simulink library "powerlib_models"  (Simulink 6.0)
settings: Solver=ode45  SolverMode=SingleTasking  StartTime=0.0  StopTime=10.0  RelTol=1e-3
values from neighbouring files (symbols this model uses):
  Ts = get(handles.edit1,'string')    [powergui.m]
undefined symbols (not defined in the file or in its folder): A, a0, a1, a2, a3, a4, a5, Ac, Amplitude, Amplitudes, B, BaseCurrent, BaseFlux, Bc, C, Capacitance, Cc, Columns, ConnectionType, Cs, ctrl, current, Current, damp, Dc, Dd, DiscIntNeverNeededParam, dref, dwo, exc, excAxis, F, Flux, fnom, Frequency, FreqVps, Gain1, gate, GH, GHd, GI, GId, GL, GLd, H, HarmonicGeneration, HT, hyd, I1_init, ib, ib2, Id1o, Inductance, InitialFlux, InitialSlope, io, Iq1o, isfinite, j, J ... (+138)
libraries: powerlib_models x32, powerlib_extras x4
(part 8 of 11)

== system powerlib_models/Discrete/asynchronous_machine/Rotor ==
  vqr,vdr : Inport  Port=1  LatchInput=off
  w-wr : Inport  Port=2  LatchInput=off
  phimq,phimd : Inport  Port=3  LatchInput=off
  1\Llr : Gain  Gain=1/Llr  SaturateOnIntegerOverflow=on
  1\Llr1 : Gain  Gain=Rr  SaturateOnIntegerOverflow=on
  1\Llr2 : Gain  Gain=1/Llr  SaturateOnIntegerOverflow=on
  1\Llr3 : Gain  Gain=Rr  SaturateOnIntegerOverflow=on
  Demux : Demux  Outputs=2
  Demux1 : Demux  Outputs=2
  Discrete-Time Integrator : DiscreteIntegrator  InitialCondition=phirqo  SampleTime=Ts  ICPrevOutput=DiscIntNeverNeededParam  ICPrevScaledInput=DiscIntNeverNeededParam
  Discrete-Time Integrator1 : DiscreteIntegrator  InitialCondition=phirdo  SampleTime=Ts  ICPrevOutput=DiscIntNeverNeededParam  ICPrevScaledInput=DiscIntNeverNeededParam
  Mux2 : Mux  Inputs=2
  Mux3 : Mux  Inputs=2
  Product : Product  SaturateOnIntegerOverflow=on  InputSameDT=on
  Product1 : Product  Orientation=left  SaturateOnIntegerOverflow=on  InputSameDT=on
  Sum1 : Sum  Inputs=++-||  SaturateOnIntegerOverflow=on  InputSameDT=on
  Sum2 : Sum  Inputs=+--  SaturateOnIntegerOverflow=on  InputSameDT=on
  Sum3 : Sum  Inputs=+-|  SaturateOnIntegerOverflow=on  InputSameDT=on
  Sum4 : Sum  Inputs=-+|  SaturateOnIntegerOverflow=on  InputSameDT=on
  web1 : Gain  Gain=web_psb  SaturateOnIntegerOverflow=on
  web_psb : Gain  Gain=web_psb  SaturateOnIntegerOverflow=on
  iqr,idr : Outport
  phiqr,phidr : Outport  Port=2
  wires:
  Mux3/1 -> phiqr,phidr/1
  Discrete-Time Integrator/1 -> Mux3/1, Product1/2, Sum3/1  "phiqr"
  web1/1 -> Discrete-Time Integrator1/1
  Sum1/1 -> web1/1
  w-wr/1 -> Product/2, Product1/1
  Product/1 -> Sum2/2
  web_psb/1 -> Discrete-Time Integrator/1
  Sum2/1 -> web_psb/1
  Discrete-Time Integrator1/1 -> Sum4/2, Product/1, Mux3/2
  vqr,vdr/1 -> Demux/1
  Product1/1 -> Sum1/1
  Demux/2 -> Sum1/2
  1\Llr3/1 -> Sum1/3
  1\Llr2/1 -> 1\Llr3/1, Mux2/2  "idr"
  Sum4/1 -> 1\Llr2/1
  Demux1/2 -> Sum4/1
  Mux2/1 -> iqr,idr/1
  1\Llr/1 -> Mux2/1, 1\Llr1/1  "iqr"
  1\Llr1/1 -> Sum2/3
  Sum3/1 -> 1\Llr/1
  Demux/1 -> Sum2/1
  Demux1/1 -> Sum3/2
  phimq,phimd/1 -> Demux1/1

== system powerlib_models/Discrete/asynchronous_machine/Stator ==
  phimq,phimd : Inport  Port=1  LatchInput=off
  vqs,vds : Inport  Port=2  LatchInput=off
  w : Inport  Port=3  LatchInput=off
  1\Llr : Gain  Gain=1/Lls  SaturateOnIntegerOverflow=on
  1\Llr1 : Gain  Gain=Rs  SaturateOnIntegerOverflow=on
  1\Llr2 : Gain  Gain=1/Lls  SaturateOnIntegerOverflow=on
  1\Llr3 : Gain  Gain=Rs  SaturateOnIntegerOverflow=on
  Demux : Demux  Outputs=2
  Demux1 : Demux  Outputs=2
  Discrete-Time Integrator : DiscreteIntegrator  InitialCondition=phisqo  SampleTime=Ts  ICPrevOutput=DiscIntNeverNeededParam  ICPrevScaledInput=DiscIntNeverNeededParam
  Discrete-Time Integrator1 : DiscreteIntegrator  InitialCondition=phisdo  SampleTime=Ts  ICPrevOutput=DiscIntNeverNeededParam  ICPrevScaledInput=DiscIntNeverNeededParam
  Mux2 : Mux  Inputs=2
  Mux3 : Mux  Inputs=2
  Mux4 : Mux  Inputs=2
  Product : Product  SaturateOnIntegerOverflow=on  InputSameDT=on
  Product1 : Product  SaturateOnIntegerOverflow=on  InputSameDT=on
  Sum1 : Sum  Inputs=++-||  SaturateOnIntegerOverflow=on  InputSameDT=on
  Sum2 : Sum  Inputs=--+  SaturateOnIntegerOverflow=on  InputSameDT=on
  Sum3 : Sum  Inputs=-+  SaturateOnIntegerOverflow=on  InputSameDT=on
  Sum4 : Sum  Inputs=+-|  SaturateOnIntegerOverflow=on  InputSameDT=on
  web1 : Gain  Gain=web_psb  SaturateOnIntegerOverflow=on
  web_psb : Gain  Gain=web_psb  SaturateOnIntegerOverflow=on
  phiqs,phids : Outport
  iqs,ids : Outport  Port=2
  phis,is : Outport  Port=3
  wires:
  phimq,phimd/1 -> Demux1/1
  Demux1/1 -> Sum4/2
  Sum4/1 -> 1\Llr/1
  1\Llr/1 -> Mux2/1, 1\Llr1/1  "iqs"
  1\Llr1/1 -> Sum2/1
  vqs,vds/1 -> Demux/1
  Sum2/1 -> web_psb/1
  Demux/1 -> Sum2/3
  Product/1 -> Sum2/2
  web_psb/1 -> Discrete-Time Integrator/1
  Discrete-Time Integrator/1 -> Mux3/1, Product1/2, Sum4/1
  Mux2/1 -> iqs,ids/1, Mux4/2
  w/1 -> Product/1, Product1/1
  Demux1/2 -> Sum3/1
  Sum3/1 -> 1\Llr2/1
  1\Llr2/1 -> 1\Llr3/1, Mux2/2  "ids"
  1\Llr3/1 -> Sum1/3
  web1/1 -> Discrete-Time Integrator1/1
  Sum1/1 -> web1/1
  Discrete-Time Integrator1/1 -> Product/2, Sum3/2, Mux3/2
  Demux/2 -> Sum1/2
  Product1/1 -> Sum1/1
  Mux3/1 -> phiqs,phids/1, Mux4/1
  Mux4/1 -> phis,is/1

== system powerlib_models/Discrete/asynchronous_machine/abc2qd ==
  v : Inport  Port=1  LatchInput=off
  sin,cos : Inport  Port=2  LatchInput=off
  1_Vb : Gain  Gain=1/Vb  SaturateOnIntegerOverflow=on
  Constant : Constant  Orientation=down  Value=ctrl==1
  Constant1 : Constant  Orientation=down  Value=ctrl==2
  Constant2 : Constant  Orientation=down  Value=ctrl==3
  Constant3 : Constant  Orientation=down  Value=ctrl
  Constant4 : Constant  Orientation=left  Value=ctrl
  Multiport Switch : MultiPortSwitch  Inputs=3  InputSameDT=on
  Multiport Switch1 : MultiPortSwitch  Inputs=3  InputSameDT=on
  Mux : Mux  Inputs=2
  Rotor reference frame : Subsystem  TreatAsAtomicUnit=on
      mask Display: disp('Rotor\nreference\nframe')
  Stationary reference frame : Subsystem  TreatAsAtomicUnit=on
      mask Display: disp('Stationary\nreference\nframe')
  Synchronous reference frame : Subsystem  TreatAsAtomicUnit=on
      mask Display: disp('Synchronous\nreference\nframe')
  transit : Subsystem
  vqr,vdr : Outport
  vqs,vds : Outport  Port=2
  wires:
  transit/1(vr,vs) -> 1_Vb/1
  Constant4/1 -> Multiport Switch1/1
  Constant3/1 -> Multiport Switch/1
  1_Vb/1 -> Mux/1
  Mux/1 -> Synchronous reference frame/1(In1), Stationary reference frame/1(In1), Rotor reference frame/1(In1)
  sin,cos/1 -> Mux/2
  Multiport Switch/1 -> vqr,vdr/1
  Synchronous reference frame/2(vqs,vds) -> Multiport Switch1/4
  Stationary reference frame/2(vqs,vds) -> Multiport Switch1/3
  Rotor reference frame/2(vqs,vds) -> Multiport Switch1/2
  Synchronous reference frame/1(vqr,vdr) -> Multiport Switch/4
  Stationary reference frame/1(vqr,vdr) -> Multiport Switch/3
  Rotor reference frame/1(vqr,vdr) -> Multiport Switch/2
  Multiport Switch1/1 -> vqs,vds/1
  Constant2/1 -> Synchronous reference frame/Enable
  Constant1/1 -> Stationary reference frame/Enable
  Constant/1 -> Rotor reference frame/Enable
  v/1 -> transit/1(vu)

== system powerlib_models/Discrete/asynchronous_machine/dq2abc ==
  sin,cos : Inport  Port=1  LatchInput=off
  iqr,idr : Inport  Port=2  LatchInput=off
  iqs,ids : Inport  Port=3  LatchInput=off
  Constant : Constant  Orientation=down  Value=ctrl==1
  Constant1 : Constant  Orientation=down  Value=ctrl==2
  Constant2 : Constant  Orientation=down  Value=ctrl==3
  Constant3 : Constant  Orientation=down  Value=ctrl
  Constant4 : Constant  Orientation=left  Value=ctrl
  Multiport Switch : MultiPortSwitch  Inputs=3  InputSameDT=on
  Multiport Switch1 : MultiPortSwitch  Inputs=3  InputSameDT=on
  Mux : Mux  Inputs=3
  Mux1 : Mux  Inputs=2
  Mux2 : Mux  Inputs=2
  Mux3 : Mux  Inputs=2
  Rotor reference frame : Subsystem  TreatAsAtomicUnit=on
      mask Display: disp('Rotor\nreference\nframe')
  Selector : Selector  Elements=elements2  InputPortWidth=4
  Stationary reference frame : Subsystem  TreatAsAtomicUnit=on
      mask Display: disp('Stationary\nreference\nframe')
  Sum2 : Sum  Inputs=-  SaturateOnIntegerOverflow=on  InputSameDT=on
  Sum3 : Sum  Inputs=-  SaturateOnIntegerOverflow=on  InputSameDT=on
  Synchronous reference frame : Subsystem  TreatAsAtomicUnit=on
      mask Display: disp('Synchronous\nreference\nframe')
  ib : Gain  Gain=ib  SaturateOnIntegerOverflow=on
  irab,isab : Outport
  irabc : Outport  Port=2
  isabc : Outport  Port=3
  wires:
  Selector/1 -> irab,isab/1
  ib/1 -> Selector/1
  Mux3/1 -> isabc/1
  Sum3/1 -> Mux3/2
  Constant4/1 -> Multiport Switch1/1
  Constant3/1 -> Multiport Switch/1
  Mux1/1 -> ib/1
  Rotor reference frame/2(isa,isb) -> Multiport Switch1/2
  sin,cos/1 -> Mux/3
  Sum2/1 -> Mux2/2
  Multiport Switch1/1 -> Mux3/1, Sum3/1, Mux1/2
  Mux2/1 -> irabc/1
  Multiport Switch/1 -> Sum2/1, Mux1/1, Mux2/1
  iqr,idr/1 -> Mux/1
  iqs,ids/1 -> Mux/2
  Mux/1 -> Synchronous reference frame/1(In1), Stationary reference frame/1(In1), Rotor reference frame/1(In1)
  Synchronous reference frame/2(isa,isb) -> Multiport Switch1/4
  Stationary reference frame/2(isa,isb) -> Multiport Switch1/3
  Synchronous reference frame/1(ira,irb) -> Multiport Switch/4
  Stationary reference frame/1(ira,irb) -> Multiport Switch/3
  Rotor reference frame/1(ira,irb) -> Multiport Switch/2
  Constant2/1 -> Synchronous reference frame/Enable
  Constant1/1 -> Stationary reference frame/Enable
  Constant/1 -> Rotor reference frame/Enable

== system powerlib_models/Discrete/asynchronous_machine/sin,cos ==
  thr,wr : Inport  Port=1  LatchInput=off
  Constant : Constant  Orientation=down  Value=ctrl<3
  Constant1 : Constant  Value=ctrl
  Constant2 : Constant  Value=0
  Constant3 : Constant  Orientation=down  Value=ctrl==3
  Constant4 : Constant  Value=ctrl
  Constant5 : Constant  Value=0
  Constant6 : Constant
  Gain : Gain  Gain=-1  SaturateOnIntegerOverflow=on
  Multiport Switch : MultiPortSwitch  Inputs=3  InputSameDT=on
  Multiport Switch1 : MultiPortSwitch  Inputs=3  InputSameDT=on
  Selector : Selector  InputPortWidth=2
  Selector1 : Selector  Elements=2  InputPortWidth=2
  Switch : Switch  Threshold=0.5  InputSameDT=on
  sin(beta),cos(beta),sin(th),cos(th) : Subsystem  TreatAsAtomicUnit=on
  sin(thr),cos(thr) : Subsystem  TreatAsAtomicUnit=on
  sin,cos : Outport
  w-wr : Outport  Port=2
  w : Outport  Port=3
  wires:
  Constant/1 -> sin(thr),cos(thr)/Enable, Switch/2
  thr,wr/1 -> Selector/1, sin(beta),cos(beta),sin(th),cos(th)/1(thr,wr), Selector1/1
  Selector/1 -> sin(thr),cos(thr)/1(thr)
  Switch/1 -> sin,cos/1
  Constant3/1 -> sin(beta),cos(beta),sin(th),cos(th)/Enable
  sin(beta),cos(beta),sin(th),cos(th)/2(we-wr) -> Multiport Switch/4
  Constant1/1 -> Multiport Switch/1
  Constant2/1 -> Multiport Switch/2
  Multiport Switch/1 -> w-wr/1
  sin(thr),cos(thr)/1(sin(thr),cos(thr)) -> Switch/1
  sin(beta),cos(beta),sin(th),cos(th)/1("sin(beta),cos(beta), sin(th),cos(th)") -> Switch/3
  Gain/1 -> Multiport Switch/3  "-wr"
  Selector1/1 -> Gain/1, Multiport Switch1/2
  Constant4/1 -> Multiport Switch1/1
  Constant5/1 -> Multiport Switch1/3
  Constant6/1 -> Multiport Switch1/4
  Multiport Switch1/1 -> w/1

== system powerlib_models/Discrete/hysteresis_transformer/Hysteresis ( always in SI ) ==
  In1 : Inport  Port=1  LatchInput=off
  Hysteresis main loop + Saturation (Lower Part) : Lookup  DialogController=Simulink.DDGSource  InputValues=LowerFlux  OutputValues=Current  SaturateOnIntegerOverflow=on
  Hysteresis main loop + Saturation. (Upper Part) : Lookup  DialogController=Simulink.DDGSource  InputValues=UpperFlux  OutputValues=Current  SaturateOnIntegerOverflow=on
  Memory : Memory
  Memory1 : Memory  Orientation=up
  SI conversion : Gain  Gain=CurrentBase  SaturateOnIntegerOverflow=on
  Selector : Selector  Elements=2  InputPortWidth=2
  Selector1 : Selector  InputPortWidth=2
  Sfunction : S-Function  FunctionName=sfun_hysteresis  Parameters=sfun_InitialFlux,HT,TransfoNumber,Ts,Tolerances,InitialSlope
  Sign : Signum
  Sum : Sum  Inputs=|+-  SaturateOnIntegerOverflow=on  InputSameDT=on
  Switch1 : Switch  InputSameDT=on
  Switch2 : Switch  Threshold=1.5  InputSameDT=on
  pu conversion : Gain  Gain=1/FluxBase  SaturateOnIntegerOverflow=on
  Out1 : Outport
  wires:
  Memory1/1 -> pu conversion/1
  Hysteresis main loop + Saturation (Lower Part)/1 -> Switch1/1
  In1/1 -> Hysteresis main loop + Saturation (Lower Part)/1, Memory/1, Sum/1, Memory1/1, Hysteresis main loop + Saturation. (Upper Part)/1
  Hysteresis main loop + Saturation. (Upper Part)/1 -> Switch1/3
  Memory/1 -> Sum/2
  Sign/1 -> Switch1/2
  pu conversion/1 -> Sfunction/1
  Sfunction/1 -> Selector/1, Selector1/1
  Switch2/1 -> Out1/1
  Switch1/1 -> Switch2/3
  Selector/1 -> Switch2/2  "Tr"
  Selector1/1 -> SI conversion/1
  SI conversion/1 -> Switch2/1  "internal loops"
  Sum/1 -> Sign/1

== system powerlib_models/Discrete/simplified_sync_mach/Subsystem ==
  i : Inport  Port=1  LatchInput=off
  v : Inport  Port=2  LatchInput=off
  e : Inport  Port=3  LatchInput=off
  theta : Inport  Port=4  LatchInput=off
  wm : Inport  Port=5  LatchInput=off
  Pe : Inport  Port=6  LatchInput=off
  Gain : Gain  Gain=[ ib2*ones(3,1); Vb3*ones(6,1); 1; Nb; Pb ]  SaturateOnIntegerOverflow=on
  Mux : Mux  Inputs=[ 3 3 3 1 1 1 ]
  * : Outport  InitialOutput=0
  wires:
  i/1 -> Mux/1
  v/1 -> Mux/2
  e/1 -> Mux/3
  theta/1 -> Mux/4
  wm/1 -> Mux/5
  Pe/1 -> Mux/6
  Mux/1 -> Gain/1
  Gain/1 -> */1

== system powerlib_models/Discrete/simplified_sync_mach/Vt ==
  note: This subsystem either converts 2 line-to-line voltages to 3 line-to-neutral voltages (internal neutral)
      | and computes floating neutral voltage or directly passes Van,Vbn,Vcn if 4-wire connection.
  V : Inport  Port=1  LatchInput=off
  1_Vb : Gain  Gain=1/Vb  SaturateOnIntegerOverflow=on
  Constant : Constant  Orientation=down  Value=ConnectionType
  Constant1 : Constant  Value=0
  Constant2 : Constant  Value=0
  Data Type  Conversion : DataTypeConversion  Orientation=left  OutDataTypeMode=boolean  SaturateOnIntegerOverflow=on  RndMeth=Zero
  Data Type  Conversion1 : DataTypeConversion  OutDataTypeMode=double  SaturateOnIntegerOverflow=on  RndMeth=Zero
  Fcn : Fcn  Expr=u[1]
  Fcn1 : Fcn  Expr=u[2]
  Fcn2 : Fcn  Expr=u[3]
  Gain : Gain  Gain=1/3  SaturateOnIntegerOverflow=on
  LL2LN : Subsystem  TreatAsAtomicUnit=on
  Logical Operator : Logic  Operator=NOT
  Mux : Mux  Inputs=2
  Mux1 : Mux  Inputs=3
  Product : Product  SaturateOnIntegerOverflow=on  InputSameDT=on
  Sum : Sum  Inputs=+  SaturateOnIntegerOverflow=on  InputSameDT=on
  Sum1 : Sum  Inputs=|++  SaturateOnIntegerOverflow=on  InputSameDT=on
  Switch2 : Switch  Threshold=0.5  InputSameDT=on
  Vn : Outport  InitialOutput=0
  Vabc : Outport  Port=2  InitialOutput=0
  wires:
  Data Type  Conversion1/1 -> Product/1
  Logical Operator/1 -> Data Type  Conversion1/1
  Data Type  Conversion/1 -> Logical Operator/1
  1_Vb/1 -> Mux/1, LL2LN/1(In1)
  V/1 -> 1_Vb/1
  Product/1 -> Sum1/2
  Mux1/1 -> Product/2
  Fcn2/1 -> Mux1/3
  Fcn1/1 -> Mux1/2
  Fcn/1 -> Mux1/1
  Mux/1 -> Fcn2/1, Fcn1/1, Fcn/1
  Constant1/1 -> Mux/2
  Sum1/1 -> Vabc/1
  LL2LN/1(Out1) -> Sum1/1, Sum/1
  Constant/1 -> Data Type  Conversion/1, LL2LN/Enable, Switch2/2
  Switch2/1 -> Vn/1
  Constant2/1 -> Switch2/3
  Gain/1 -> Switch2/1
  Sum/1 -> Gain/1

== system powerlib_models/Discrete/simplified_sync_mach/Z ==
  note: This subsystem models the internal impedance of
      | the machine, which consists of  a series RL circuit.
  e : Inport  Port=1  LatchInput=off
  v : Inport  Port=2  LatchInput=off
  1/L : Gain  Gain=web_psb/L  SaturateOnIntegerOverflow=on
  Discrete-Time Integrator : DiscreteIntegrator  IntegratorMethod=Integration: Trapezoidal  InitialCondition=io  SampleTime=Ts  ICPrevOutput=DiscIntNeverNeededParam  ICPrevScaledInput=DiscIntNeverNeededParam
  R : Gain  Orientation=left  Gain=R  SaturateOnIntegerOverflow=on
  Sum5 : Sum  Inputs=-+-  SaturateOnIntegerOverflow=on  InputSameDT=on
  Unit Delay : UnitDelay  X0=io  SampleTime=Ts
  i : Outport  InitialOutput=0
  wires:
  e/1 -> Sum5/2
  R/1 -> Sum5/1
  Sum5/1 -> 1/L/1
  v/1 -> Sum5/3
  1/L/1 -> Discrete-Time Integrator/1
  Discrete-Time Integrator/1 -> Unit Delay/1
  Unit Delay/1 -> R/1, i/1

== system powerlib_models/Discrete/simplified_sync_mach/gen ==
  note: This subsystem generates the 3 line-to-neutral voltages inside the machine.
  theta : Inport  Port=1  LatchInput=off
  E : Inport  Port=2  LatchInput=off
  Vn : Inport  Port=3  LatchInput=off
  1_Vb2 : Gain  Gain=1/Vb2  SaturateOnIntegerOverflow=on
  Mux : Mux  Inputs=3
  Product : Product  SaturateOnIntegerOverflow=on  InputSameDT=on
  Sum : Sum  Inputs=|++  SaturateOnIntegerOverflow=on  InputSameDT=on
  Sum1 : Sum  Orientation=down  Inputs=--  SaturateOnIntegerOverflow=on  InputSameDT=on
  rem(wt,2pi) : Fcn  Expr=rem(u[1],2*pi)
  sin(a) : Fcn  Expr=sin(u)
  sin(b) : Fcn  Expr=sin(u-pi23)
  e : Outport  InitialOutput=0
  wires:
  Sum/1 -> e/1
  Product/1 -> Sum/1
  Mux/1 -> Product/1
  Vn/1 -> Sum/2
  1_Vb2/1 -> Product/2
  E/1 -> 1_Vb2/1
  sin(b)/1 -> Mux/2, Sum1/1
  Sum1/1 -> Mux/3
  sin(a)/1 -> Mux/1, Sum1/2
  theta/1 -> rem(wt,2pi)/1
  rem(wt,2pi)/1 -> sin(b)/1, sin(a)/1

== system powerlib_models/Discrete/simplified_sync_mach/wattmeter ==
  note: This subsystem computes the total electrical
      | power delivered or absorbed by the machine.
  i : Inport  Port=1  LatchInput=off
  v : Inport  Port=2  LatchInput=off
  2_3 : Gain  Gain=2/3  SaturateOnIntegerOverflow=on
  Product : Product  SaturateOnIntegerOverflow=on  InputSameDT=on
  Sum : Sum  Inputs=+  SaturateOnIntegerOverflow=on  InputSameDT=on
  Pe : Outport  InitialOutput=0
  wires:
  2_3/1 -> Pe/1
  Sum/1 -> 2_3/1
  v/1 -> Product/2
  i/1 -> Product/1
  Product/1 -> Sum/1

== system powerlib_models/Discrete/synchronous_machine/Delta angle ==
  Vq : Inport  Port=1  PortDimensions=1  LatchInput=off
  Vd : Inport  Port=2  PortDimensions=1  LatchInput=off
  Cartesian to Polar : Subsystem
      mask Type: Cart2Polar
      mask Description:
      | Transformation from cartesian to polar coordinates.
      | [x, y] -> [r, theta]
      | 
      | r = sqrt(x^2 + y^2);
      | theta = atan(y/x);
      mask Help: Unmask this block for more help.
      mask Display: plot(0,0,100,100,[24,20,15,20,20],[85,95,85,95,20],[80,20,95,85,95,85],[70,20,20,15,20,24],[56,56,55,52,50,46],[20,26,31,35,38,42])
  Radians to Degrees : Subsystem
      mask Type: RadiansToDegrees
      mask Description:
      | Conversion from Radians to Degrees.
      | 
      | D=180/pi*R
      mask Help: This block converts from Radians to Degrees.
      mask Display: disp('R2D')
  Terminator2 : Terminator
  delta : Outport
  wires:
  Vd/1 -> Cartesian to Polar/2(y)
  Radians to Degrees/1(Degrees out) -> delta/1  "delta"
  Vq/1 -> Cartesian to Polar/1(x)
  Cartesian to Polar/1(r) -> Terminator2/1
  Cartesian to Polar/2(theta) -> Radians to Degrees/1(Radians in)

== system powerlib_models/Discrete/synchronous_machine/PQ ==
  note: P = Vd*Id + Vq*Iq
  note: Q = Vq*Id-Vd*Iq
  note: PQ Measurement:
  Vq : Inport  Port=1  PortDimensions=1  LatchInput=off
  Vd : Inport  Port=2  PortDimensions=1  LatchInput=off
  Iq : Inport  Port=3  PortDimensions=2  LatchInput=off
  Demux1 : Demux  Outputs=[1,1]
  Gain : Gain  Gain=Gain1  SaturateOnIntegerOverflow=on
  Gain1 : Gain  Gain=Gain1  SaturateOnIntegerOverflow=on
  Product{2..5} (4 alike) : Product  SaturateOnIntegerOverflow=on  InputSameDT=on
  Sum : Sum  SaturateOnIntegerOverflow=on  InputSameDT=on
  Sum1 : Sum  Inputs=+-  SaturateOnIntegerOverflow=on  InputSameDT=on
  Peo : Outport
  Qeo : Outport  Port=2
  wires:
  Demux1/1 -> Product5/2, Product2/2
  Iq/1 -> Demux1/1
  Gain1/1 -> Qeo/1
  Gain/1 -> Peo/1
  Product2/1 -> Sum/1
  Product3/1 -> Sum/2
  Product4/1 -> Sum1/1
  Product5/1 -> Sum1/2
  Sum/1 -> Gain/1  "Peo"
  Sum1/1 -> Gain1/1  "Qeo"
  Vd/1 -> Product3/1, Product5/1
  Vq/1 -> Product2/1, Product4/1
  Demux1/2 -> Product3/2, Product4/2

== system powerlib_models/Discrete/synchronous_machine/Vfd ==
  Vf : Inport  Port=1  LatchInput=off
  Constant : Constant  Value=excAxis
  Ground2 : Ground
  Switch : Switch  Threshold=1.5  InputSameDT=on
  Switch1 : Switch  Threshold=1.5  InputSameDT=on
  Vkq1 : Outport
  Vfd : Outport  Port=2
  wires:
  Switch/1 -> Vkq1/1
  Switch1/1 -> Vfd/1
  Constant/1 -> Switch1/2, Switch/2
  Vf/1 -> Switch/1, Switch1/3
  Ground2/1 -> Switch/3, Switch1/1

== system powerlib_models/Discrete/synchronous_machine/abc2qd ==
  note: This subsystem converts Vab and Vbc to Vd,Vq. The sine and cosine com-
      | puted here are sent to the inverse transformation subsystem qd/abc.
  v : Inport  Port=1  LatchInput=off
  theta : Inport  Port=2  LatchInput=off
  1_Vb : Gain  Gain=1/Vb  SaturateOnIntegerOverflow=on
  Elementary Math : ElementaryMath
  Elementary Math1 : ElementaryMath  Operator=cos
  Fcn2 : Fcn  Expr=(u[4]*(2*u[1]+u[2]) + (sqrt3*u[2]*u[3])) * one_third
  Fcn3 : Fcn  Expr=(u[3]*(2*u[1]+u[2]) + (-sqrt3*u[2]*u[4])) * one_third
  Mux1 : Mux  Inputs=[ 2 2 ]
  Mux2 : Mux  Orientation=down  Inputs=[ 1 1 ]
  Mux3 : Mux  Inputs=2
  cos,sin : Outport  InitialOutput=0
  vq : Outport  Port=2  InitialOutput=0
  vd : Outport  Port=3  InitialOutput=0
  vq,vd : Outport  Port=4  InitialOutput=0
  wires:
  Fcn3/1 -> Mux2/2, vd/1
  Fcn2/1 -> Mux2/1, vq/1
  Elementary Math1/1 -> Mux3/2
  Elementary Math/1 -> Mux3/1
  theta/1 -> Elementary Math1/1, Elementary Math/1
  Mux3/1 -> cos,sin/1, Mux1/2
  Mux1/1 -> Fcn3/1, Fcn2/1
  v/1 -> 1_Vb/1
  1_Vb/1 -> Mux1/1
  Mux2/1 -> vq,vd/1

== system powerlib_models/Discrete/synchronous_machine/currents and mutual fluxes ==
  note: This subsystem computes the mutual fluxes phimd
      | and phimq and all direct and quadrature axis
      | currents in the model.
  phiq : Inport  Port=1  LatchInput=off
  phikq2 : Inport  Port=2  LatchInput=off
  phid : Inport  Port=3  LatchInput=off
  phifd : Inport  Port=4  LatchInput=off
  phikq1 : Inport  Port=5  LatchInput=off
  phikd : Inport  Port=6  LatchInput=off
  -1_Ll : Gain  Gain=-1/Ll  SaturateOnIntegerOverflow=on
  "-1_Ll " : Gain  Gain=-1/Ll  SaturateOnIntegerOverflow=on
  1_Llfd : Gain  Gain=1/Llfd  SaturateOnIntegerOverflow=on
  1_Llkd : Gain  Gain=1/Llkd  SaturateOnIntegerOverflow=on
  1_Llkq1 : Gain  Gain=1/Llkq1  SaturateOnIntegerOverflow=on
  1_Llkq2 : Gain  Gain=1/Llkq2  SaturateOnIntegerOverflow=on
  Lad_Ll : Gain  Gain=Lad/Ll  SaturateOnIntegerOverflow=on
  Lad_Llfd : Gain  Gain=Lad/Llfd  SaturateOnIntegerOverflow=on
  Lad_Llkd : Gain  Gain=Lad/Llkd  SaturateOnIntegerOverflow=on
  Laq_Ll : Gain  Gain=Laq/Ll  SaturateOnIntegerOverflow=on
  Laq_Llkq1 : Gain  Gain=Laq/Llkq1  SaturateOnIntegerOverflow=on
  Laq_Llkq2 : Gain  Gain=Laq/Llkq2  SaturateOnIntegerOverflow=on
  Mux1 : Mux  Inputs=2
  Mux3 : Mux  Inputs=[2 1 1 1 1 1 1]
  Saturation : Subsystem
  Sum{17..22} (6 alike) : Sum  Inputs=-+  SaturateOnIntegerOverflow=on  InputSameDT=on
  sum : Sum  Inputs=+++  SaturateOnIntegerOverflow=on  InputSameDT=on
  sum1 : Sum  Inputs=+++  SaturateOnIntegerOverflow=on  InputSameDT=on
  phimq : Outport  InitialOutput=0
  "iq,id,ifd, ikq1,ikq2,ikd, phimq,phimd" : Outport  Port=2  InitialOutput=0
  iq,id : Outport  Port=3  InitialOutput=0
  phimd : Outport  Port=4  InitialOutput=0
  wires:
  phikq1/1 -> Sum18/2, Laq_Llkq1/1
  phikq2/1 -> Sum22/2, Laq_Llkq2/1
  Laq_Llkq1/1 -> sum/2
  Laq_Llkq2/1 -> sum/3
  Laq_Ll/1 -> sum/1
  phiq/1 -> Sum17/2, Laq_Ll/1
  phikd/1 -> Sum19/2, Lad_Llkd/1
  phid/1 -> Lad_Ll/1, Sum20/2
  phifd/1 -> Sum21/2, Lad_Llfd/1
  Lad_Ll/1 -> sum1/1
  Lad_Llfd/1 -> sum1/2
  Lad_Llkd/1 -> sum1/3
  Mux1/1 -> Mux3/1, iq,id/1
  -1_Ll/1 -> Mux1/1  "iq"
  Sum22/1 -> 1_Llkq2/1
  Sum17/1 -> -1_Ll/1
  Sum18/1 -> 1_Llkq1/1
  1_Llkd/1 -> Mux3/5  "ikd"
  1_Llfd/1 -> Mux3/2  "ifd"
  Sum19/1 -> 1_Llkd/1
  Sum21/1 -> 1_Llfd/1
  "-1_Ll "/1 -> Mux1/2  "id"
  Sum20/1 -> "-1_Ll "/1
  1_Llkq1/1 -> Mux3/3  "ikq1"
  1_Llkq2/1 -> Mux3/4  "ikq2"
  Mux3/1 -> "iq,id,ifd, ikq1,ikq2,ikd, phimq,phimd"/1
  sum/1 -> Saturation/1(phimq_in)  "phimq"
  sum1/1 -> Saturation/2(phimd_in)  "phimd"
  Saturation/1(phimq_out) -> phimq/1, Sum18/1, Sum22/1, Mux3/6, Sum17/1
  Saturation/2(phimd_out) -> phimd/1, Sum20/1, Sum21/1, Sum19/1, Mux3/7

== system powerlib_models/Discrete/synchronous_machine/phid ==
  note: This subsystem computes the direct axis flux phid.
  w : Inport  Port=1  LatchInput=off
  phiq : Inport  Port=2  LatchInput=off
  vd : Inport  Port=3  LatchInput=off
  phimd : Inport  Port=4  LatchInput=off
  Discrete-Time Integrator : DiscreteIntegrator  IntegratorMethod=Integration: Trapezoidal  InitialCondition=phido  SampleTime=Ts  ICPrevOutput=DiscIntNeverNeededParam  ICPrevScaledInput=DiscIntNeverNeededParam
  Product1 : Product  SaturateOnIntegerOverflow=on  InputSameDT=on
  Rs_Ll : Gain  Gain=Rs/Ll  SaturateOnIntegerOverflow=on
  Sum2 : Sum  Inputs=+++  SaturateOnIntegerOverflow=on  InputSameDT=on
  Sum9 : Sum  Inputs=+-  SaturateOnIntegerOverflow=on  InputSameDT=on
  Unit Delay1 : UnitDelay  X0=phido  SampleTime=Ts
  web_psb : Gain  Gain=web_psb  SaturateOnIntegerOverflow=on
  phid : Outport  InitialOutput=0
  wires:
  Discrete-Time Integrator/1 -> Unit Delay1/1
  web_psb/1 -> Discrete-Time Integrator/1
  Sum2/1 -> web_psb/1
  Rs_Ll/1 -> Sum2/3
  Sum9/1 -> Rs_Ll/1
  Product1/1 -> Sum2/1
  w/1 -> Product1/1
  phiq/1 -> Product1/2
  vd/1 -> Sum2/2
  phimd/1 -> Sum9/1
  Unit Delay1/1 -> phid/1, Sum9/2

== system powerlib_models/Discrete/synchronous_machine/phifd ==
  note: This subsystem computes the field flux phifd.
  vfd : Inport  Port=1  LatchInput=off
  phimd : Inport  Port=2  LatchInput=off
  Discrete-Time Integrator : DiscreteIntegrator  IntegratorMethod=Integration: Trapezoidal  InitialCondition=phifdo  SampleTime=Ts  ICPrevOutput=DiscIntNeverNeededParam  ICPrevScaledInput=DiscIntNeverNeededParam
  N : Gain  Gain=N  SaturateOnIntegerOverflow=on
  Rf_Llfd : Gain  Gain=Rf/Llfd  SaturateOnIntegerOverflow=on
  Sum10 : Sum  Inputs=+-  SaturateOnIntegerOverflow=on  InputSameDT=on
  Sum3 : Sum  SaturateOnIntegerOverflow=on  InputSameDT=on
  Unit Delay : UnitDelay  Orientation=left  X0=phifdo  SampleTime=Ts
  web_psb : Gain  Gain=web_psb  SaturateOnIntegerOverflow=on
  phifd : Outport  InitialOutput=0
  wires:
  Sum3/1 -> web_psb/1
  Discrete-Time Integrator/1 -> phifd/1, Unit Delay/1
  web_psb/1 -> Discrete-Time Integrator/1
  phimd/1 -> Sum10/1
  Sum10/1 -> Rf_Llfd/1
  Rf_Llfd/1 -> Sum3/2
  vfd/1 -> N/1
  N/1 -> Sum3/1
  Unit Delay/1 -> Sum10/2

== system powerlib_models/Discrete/synchronous_machine/phikd ==
  note: This subsystem computes the direct axis damper flux phikd.
  phimd : Inport  Port=1  LatchInput=off
  vkd : Inport  Port=2  LatchInput=off
  Discrete-Time Integrator : DiscreteIntegrator  IntegratorMethod=Integration: Trapezoidal  InitialCondition=phikdo  SampleTime=Ts  ICPrevOutput=DiscIntNeverNeededParam  ICPrevScaledInput=DiscIntNeverNeededParam
  Rkd_Llkd : Gain  Gain=Rkd/Llkd  SaturateOnIntegerOverflow=on
  Sum11 : Sum  Inputs=-+  SaturateOnIntegerOverflow=on  InputSameDT=on
  Sum4 : Sum  SaturateOnIntegerOverflow=on  InputSameDT=on
  Unit Delay : UnitDelay  Orientation=left  X0=phikdo  SampleTime=Ts
  web_psb : Gain  Gain=web_psb  SaturateOnIntegerOverflow=on
  phikd : Outport  InitialOutput=0
  wires:
  Sum4/1 -> web_psb/1
  Discrete-Time Integrator/1 -> phikd/1, Unit Delay/1
  web_psb/1 -> Discrete-Time Integrator/1
  vkd/1 -> Sum4/2
  phimd/1 -> Sum11/2
  Sum11/1 -> Rkd_Llkd/1
  Rkd_Llkd/1 -> Sum4/1
  Unit Delay/1 -> Sum11/1

== system powerlib_models/Discrete/synchronous_machine/phikq1 ==
  note: This subsystem computes the quadrature axis damper flux phikq.
  phimq : Inport  Port=1  LatchInput=off
  vkq1 : Inport  Port=2  LatchInput=off
  Discrete-Time Integrator : DiscreteIntegrator  IntegratorMethod=Integration: Trapezoidal  InitialCondition=phikq1o  SampleTime=Ts  ICPrevOutput=DiscIntNeverNeededParam  ICPrevScaledInput=DiscIntNeverNeededParam
  Rkq1_Llkq1 : Gain  Gain=Rkq1/Llkq1  SaturateOnIntegerOverflow=on
  Sum1 : Sum  SaturateOnIntegerOverflow=on  InputSameDT=on
  Sum7 : Sum  Inputs=-+  SaturateOnIntegerOverflow=on  InputSameDT=on
  Unit Delay : UnitDelay  Orientation=left  X0=phikq1o  SampleTime=Ts
  web_psb : Gain  Gain=web_psb  SaturateOnIntegerOverflow=on
  phikq1 : Outport  InitialOutput=0
  wires:
  Rkq1_Llkq1/1 -> Sum1/1
  Sum7/1 -> Rkq1_Llkq1/1
  Sum1/1 -> web_psb/1
  phimq/1 -> Sum7/2
  vkq1/1 -> Sum1/2
  web_psb/1 -> Discrete-Time Integrator/1
  Discrete-Time Integrator/1 -> phikq1/1, Unit Delay/1
  Unit Delay/1 -> Sum7/1

== system powerlib_models/Discrete/synchronous_machine/phikq2 ==
  note: This subsystem computes the quadrature axis damper flux phikq2.
  vkq2 : Inport  Port=1  LatchInput=off
  phimq : Inport  Port=2  LatchInput=off
  Enabled integrator : Subsystem  TreatAsAtomicUnit=on
      mask Display: disp('1/s')
  Rkq2_Llkq2 : Gain  Gain=Rkq2/Llkq2  SaturateOnIntegerOverflow=on
  Sum1 : Sum  SaturateOnIntegerOverflow=on  InputSameDT=on
  Sum7 : Sum  Inputs=-+  SaturateOnIntegerOverflow=on  InputSameDT=on
  Unit Delay : UnitDelay  Orientation=left  X0=phikq2o  SampleTime=Ts
  web_psb : Gain  Gain=web_psb  SaturateOnIntegerOverflow=on
  wref : Constant  Value=isfinite(Llkq2)
  phikq2 : Outport  InitialOutput=0
  wires:
  phimq/1 -> Sum7/2
  Sum1/1 -> web_psb/1
  Rkq2_Llkq2/1 -> Sum1/1
  vkq2/1 -> Sum1/2
  Sum7/1 -> Rkq2_Llkq2/1
  web_psb/1 -> Enabled integrator/1(In1)
  Enabled integrator/1(Out1) -> phikq2/1, Unit Delay/1
  wref/1 -> Enabled integrator/Enable
  Unit Delay/1 -> Sum7/1

== system powerlib_models/Discrete/synchronous_machine/phiq ==
  note: This subsystem computes the quadrature axis flux phiq.
  vq : Inport  Port=1  LatchInput=off
  w : Inport  Port=2  LatchInput=off
  phid : Inport  Port=3  LatchInput=off
  phimq : Inport  Port=4  LatchInput=off
  Discrete-Time Integrator : DiscreteIntegrator  IntegratorMethod=Integration: Trapezoidal  InitialCondition=phiqo  SampleTime=Ts  ICPrevOutput=DiscIntNeverNeededParam  ICPrevScaledInput=DiscIntNeverNeededParam
  Product2 : Product  SaturateOnIntegerOverflow=on  InputSameDT=on
  Rs_Ll : Gain  Gain=Rs/Ll  SaturateOnIntegerOverflow=on
  Sum : Sum  Inputs=+-+  SaturateOnIntegerOverflow=on  InputSameDT=on
  Sum6 : Sum  Inputs=+-  SaturateOnIntegerOverflow=on  InputSameDT=on
  Unit Delay1 : UnitDelay  X0=phiqo  SampleTime=Ts
  web_psb : Gain  Gain=web_psb  SaturateOnIntegerOverflow=on
  phiq : Outport  InitialOutput=0
  wires:
  Discrete-Time Integrator/1 -> Unit Delay1/1
  web_psb/1 -> Discrete-Time Integrator/1
  phimq/1 -> Sum6/1
  phid/1 -> Product2/2
  w/1 -> Product2/1
  vq/1 -> Sum/1
  Product2/1 -> Sum/2
  Sum6/1 -> Rs_Ll/1
  Rs_Ll/1 -> Sum/3
  Sum/1 -> web_psb/1
  Unit Delay1/1 -> phiq/1, Sum6/2

== system powerlib_models/Discrete/synchronous_machine/qd2abc ==
  note: This subsystem converts id,iq to ia,ib,ic.
  sin,cos : Inport  Port=1  LatchInput=off
  iq,id : Inport  Port=2  LatchInput=off
  Fcn : Fcn  Expr=u[3]*u[2] + u[4]*u[1]
  Fcn1 : Fcn  Expr=(u[2]*(-u[3]-sqrt3*u[4]) + u[1]*(sqrt3*u[3]-u[4]))*0.5
  Mux : Mux  Inputs=[ 2 2 ]
  Mux1_ : Mux  Inputs=3
  Sum : Sum  Orientation=down  Inputs=--  SaturateOnIntegerOverflow=on  InputSameDT=on
  ib : Gain  Gain=ib  SaturateOnIntegerOverflow=on
  is(A) : Outport  InitialOutput=0
  is(pu) : Outport  Port=2  InitialOutput=0
  wires:
  ib/1 -> is(A)/1
  Fcn1/1 -> Sum/2, Mux1_/2
  Fcn/1 -> Mux1_/1, Sum/1
  Sum/1 -> Mux1_/3
  Mux1_/1 -> ib/1, is(pu)/1
  Mux/1 -> Fcn/1, Fcn1/1
  sin,cos/1 -> Mux/1
  iq,id/1 -> Mux/2

== system powerlib_models/Phasors/3_Phase_Prog_Source/Seq A Generation ==
  Enable : Inport  Port=1  LatchInput=off
  Gain3 : Gain  Gain=pi/180  SaturateOnIntegerOverflow=on
  Magnitude-Angle to Complex : MagnitudeAngleToComplex
  Multiport Switch : MultiPortSwitch  Inputs=3  InputSameDT=on
  Negative-sequence : Constant  Value=[0 2*pi/3 -2*pi/3]
  Phase_Harmo : Constant  Value=Phase_Harmo
  Phase_Harmo1 : Constant  Value=Mag_Harmo
  Phase_Harmo2 : Constant  Value=Seq_Harmo
  Positive-sequence : Constant  Value=[0 -2*pi/3 2*pi/3]
  Product1 : Product  SaturateOnIntegerOverflow=on  InputSameDT=on
  Sum : Sum  SaturateOnIntegerOverflow=on  InputSameDT=on
  Sum1 : Sum  SaturateOnIntegerOverflow=on  InputSameDT=on
  Zero-sequence : Constant  Value=[0 0 0]
  valp_nom2 : Constant
  Seq120 : Outport
  wires:
  Enable/1 -> Product1/1
  Phase_Harmo1/1 -> Magnitude-Angle to Complex/1
  Multiport Switch/1 -> Sum/2
  Phase_Harmo/1 -> Gain3/1
  valp_nom2/1 -> Sum1/2
  Phase_Harmo2/1 -> Sum1/1
  Sum1/1 -> Multiport Switch/1
  Product1/1 -> Seq120/1
  Magnitude-Angle to Complex/1 -> Product1/2
  Gain3/1 -> Sum/1
  Negative-sequence/1 -> Multiport Switch/4
  Positive-sequence/1 -> Multiport Switch/3
  Zero-sequence/1 -> Multiport Switch/2
  Sum/1 -> Magnitude-Angle to Complex/2

== system powerlib_models/Phasors/3_Phase_Prog_Source/Seq B Generation ==
  Enable : Inport  Port=1  LatchInput=off
  Gain3 : Gain  Gain=pi/180  SaturateOnIntegerOverflow=on
  Magnitude-Angle to Complex : MagnitudeAngleToComplex
  Multiport Switch : MultiPortSwitch  Inputs=3  InputSameDT=on
  Negative-sequence : Constant  Value=[0 2*pi/3 -2*pi/3]
  Phase_Harmo : Constant  Value=Phase_Harmo
  Phase_Harmo1 : Constant  Value=Mag_Harmo
  Phase_Harmo2 : Constant  Value=Seq_Harmo
  Positive-sequence : Constant  Value=[0 -2*pi/3 2*pi/3]
  Product1 : Product  SaturateOnIntegerOverflow=on  InputSameDT=on
  Sum : Sum  SaturateOnIntegerOverflow=on  InputSameDT=on
  Sum1 : Sum  SaturateOnIntegerOverflow=on  InputSameDT=on
  Zero-sequence : Constant  Value=[0 0 0]
  valp_nom2 : Constant
  Seq120 : Outport
  wires:
  Sum/1 -> Magnitude-Angle to Complex/2
  Zero-sequence/1 -> Multiport Switch/2
  Positive-sequence/1 -> Multiport Switch/3
  Negative-sequence/1 -> Multiport Switch/4
  Gain3/1 -> Sum/1
  Magnitude-Angle to Complex/1 -> Product1/2
  Product1/1 -> Seq120/1
  Sum1/1 -> Multiport Switch/1
  Phase_Harmo2/1 -> Sum1/1
  valp_nom2/1 -> Sum1/2
  Phase_Harmo/1 -> Gain3/1
  Multiport Switch/1 -> Sum/2
  Phase_Harmo1/1 -> Magnitude-Angle to Complex/1
  Enable/1 -> Product1/1

== system powerlib_models/Phasors/3_Phase_Prog_Source/Timer ==
  Clock : Clock
  Look-Up Table : Lookup  DialogController=Simulink.DDGSource  InputValues=tv  OutputValues=opv  SaturateOnIntegerOverflow=on
  Out : Outport
  wires:
  Clock/1 -> Look-Up Table/1
  Look-Up Table/1 -> Out/1

== system powerlib_models/Phasors/3_Phase_Prog_Source/Variation SubSystem ==
  VariationType : Inport  Port=1  LatchInput=off
  Constant : Constant  Value=2
  Constant1 : Constant  Value=0
  Constant2 : Constant
  Constant3 : Constant
  Constant4 : Constant  Value=0
  Constant5 : Constant  Value=0
  Data Type  Conversion1 : DataTypeConversion  OutDataTypeMode=boolean  SaturateOnIntegerOverflow=on  RndMeth=Zero
  Data Type  Conversion2 : DataTypeConversion  Orientation=up  OutDataTypeMode=boolean  SaturateOnIntegerOverflow=on  RndMeth=Zero
  Gain1 : Gain  Gain=2*pi  SaturateOnIntegerOverflow=on
  Integrator : Integrator
  Logical Operator : Logic
  Logical Operator1 : Logic  Orientation=up  Operator=NOT
  Memory : Memory  Orientation=left
  Multiport Switch1 : MultiPortSwitch  InputSameDT=on
  Product : Product  SaturateOnIntegerOverflow=on  InputSameDT=on
  Product1 : Product  SaturateOnIntegerOverflow=on  InputSameDT=on
  Product2 : Product  SaturateOnIntegerOverflow=on  InputSameDT=on
  Relational Operator : RelationalOperator  Operator===  InputSameDT=on
  Relational Operator1 : RelationalOperator  Operator===  InputSameDT=on
  Step : Step  Time=Ton_Variation  SampleTime=0
  Step1 : Step  Time=Toff_Variation  Before=1  After=0  SampleTime=0
  Switch{,1..3} (4 alike) : Switch  Threshold=0.5  InputSameDT=on
  Trigonometric Function1 : Trigonometry
  valp_nom6 : Constant  Value=VariationStep
  valp_nom7 : Constant  Value=VariationRate
  valp_nom8 : Constant  Value=VariationMag
  valp_nom9 : Constant  Value=VariationFreq
  Value : Outport
  wires:
  Relational Operator1/1 -> Data Type  Conversion1/1
  Data Type  Conversion2/1 -> Logical Operator1/1
  Trigonometric Function1/1 -> Product/2
  valp_nom8/1 -> Product/1
  valp_nom9/1 -> Gain1/1
  Gain1/1 -> Product1/2
  Product1/1 -> Trigonometric Function1/1
  Product/1 -> Multiport Switch1/4  "Mod"
  valp_nom7/1 -> Switch1/1
  Constant2/1 -> Switch1/3
  Constant4/1 -> Switch/3
  Switch1/1 -> Switch/1
  Constant/1 -> Relational Operator/2
  Switch/1 -> Integrator/1
  Relational Operator/1 -> Switch1/2
  valp_nom6/1 -> Product2/1
  Product2/1 -> Multiport Switch1/2  "Step"
  Integrator/1 -> Product1/1, Multiport Switch1/3  "Ramp"
  VariationType/1 -> Multiport Switch1/1, Relational Operator1/1, Relational Operator/1
  Step/1 -> Switch/2, Product2/2  "Ton"
  Multiport Switch1/1 -> Switch2/1
  Memory/1 -> Switch2/3
  Constant1/1 -> Switch3/1
  Switch2/1 -> Memory/1, Switch3/3
  Switch3/1 -> Value/1
  Constant3/1 -> Relational Operator1/2
  Step1/1 -> Data Type  Conversion2/1, Switch2/2  "Toff"
  Logical Operator/1 -> Switch3/2
  Logical Operator1/1 -> Logical Operator/1
  Constant5/1 -> Multiport Switch1/5
  Data Type  Conversion1/1 -> Logical Operator/2

== system powerlib_models/Phasors/Dynamic_Load/Break  Alg. Loop I1 ==
  In : Inport  Orientation=left  Port=1  LatchInput=off
  Complex to Real-Imag : ComplexToRealImag  Orientation=left
  Real-Imag to Complex : RealImagToComplex  Orientation=left
  imag : Subsystem  Orientation=left  mask(Transfer Function with Initial Outputs){N=[1], D=[100e-6  1], Y0=imag(I1_init), U0=imag(I1_init)}
      mask prompts: N "Numerator:"; D "Denominator:"; Y0 "Initial output:"; U0 "Initial input:"
      mask help: Vector expressions for numerator, and denominator. Coefficients are in descending powers of s.
      mask init:
      | [A,B,C,Dd]=tf2ss(N,D);if (isempty(Y0));[m,n]=size(A);X0=zeros(1,m); end; if (isempty(U0));[m,p]=size(B);U0=zeros(1,p);end;X0=getxo(A,B,C,Dd,U0,Y0,0);
      mask Help: Specify the initial output for the transfer function.  An optimization routine attempts to determine the appropriate initial states so that the specified initial output is achieved.  For more details, see the m-file getxo.m
      mask Display: dpoly(N,D,'s')
  real : Subsystem  Orientation=left  mask(Transfer Function with Initial Outputs){N=[1], D=[100e-6  1], Y0=real(I1_init), U0=real(I1_init)}
      mask prompts: N "Numerator:"; D "Denominator:"; Y0 "Initial output:"; U0 "Initial input:"
      mask help: Vector expressions for numerator, and denominator. Coefficients are in descending powers of s.
      mask init:
      | [A,B,C,Dd]=tf2ss(N,D);if (isempty(Y0));[m,n]=size(A);X0=zeros(1,m); end; if (isempty(U0));[m,p]=size(B);U0=zeros(1,p);end;X0=getxo(A,B,C,Dd,U0,Y0,0);
      mask Help: Specify the initial output for the transfer function.  An optimization routine attempts to determine the appropriate initial states so that the specified initial output is achieved.  For more details, see the m-file getxo.m
      mask Display: dpoly(N,D,'s')
  Out : Outport  Orientation=left
  wires:
  imag/1(Out1) -> Real-Imag to Complex/2
  Complex to Real-Imag/2 -> imag/1(In1)
  real/1(Out1) -> Real-Imag to Complex/1
  Complex to Real-Imag/1 -> real/1(In1)
  Real-Imag to Complex/1 -> Out/1
  In/1 -> Complex to Real-Imag/1

== system powerlib_models/Phasors/Dynamic_Load/I1  ==
  note: V2= 1/3(Vab -a*Vbc)
  note: V1= 1/3(Vab -a^2*Vbc)
  note: I1= (S/V1)'
  Vab Vbc cmplx : Inport  Port=1  LatchInput=off
  S=P+jQ : Inport  Port=2  LatchInput=off
  (a^2)/3 : Gain  Gain=1/3*exp(-j*2*pi/3)  SaturateOnIntegerOverflow=on
  Complex to Magnitude-Angle : ComplexToMagnitudeAngle  Output=Magnitude
  Conj1 : Math  Operator=conj  SaturateOnIntegerOverflow=on
  Demux : Demux  Outputs=2
  Gain : Gain  Gain=1/3  SaturateOnIntegerOverflow=on
  Product : Product  Inputs=/*  SaturateOnIntegerOverflow=on  InputSameDT=on
  Sum3 : Sum  Inputs=+-  SaturateOnIntegerOverflow=on  InputSameDT=on
  pu>V : Gain  Orientation=down  Gain=Vnom*sqrt(3)/sqrt(2)  SaturateOnIntegerOverflow=on
  |V1| : Outport
  I1 : Outport  Port=2
  wires:
  (a^2)/3/1 -> Sum3/2
  Demux/2 -> (a^2)/3/1
  Gain/1 -> Sum3/1
  Vab Vbc cmplx/1 -> Demux/1
  Demux/1 -> Gain/1
  Sum3/1 -> Complex to Magnitude-Angle/1, pu>V/1  "V1"
  Complex to Magnitude-Angle/1 -> |V1|/1
  S=P+jQ/1 -> Product/2
  Product/1 -> Conj1/1
  Conj1/1 -> I1/1
  pu>V/1 -> Product/1

== system powerlib_models/Phasors/Dynamic_Load/Phase currents ==
  note: Ib= a^2*I1
  note: Ia= I1
  I1 : Inport  Port=1  LatchInput=off
  Mux1 : Mux  Inputs=2
  a^2 : Gain  Gain=exp(-j*2*pi/3)  SaturateOnIntegerOverflow=on
  Ia Ib cmplx : Outport
  wires:
  Mux1/1 -> Ia Ib cmplx/1  "ia ib"
  I1/1 -> a^2/1, Mux1/1
  a^2/1 -> Mux1/2

== system powerlib_models/Phasors/Dynamic_Load/Power ==
  note: V>Vmin :
      |
      |    P=Po*(V/Vo)^np
      |    Q=Qo*(V/Vo)^np
  note: V<Vmin
      | Constant impedance load :
      |
      |  P=Po*kp*V^2
      | Q=Qo*kq*V^2
  note: kp=Vmin^(np-2)/Vo^np
      | kq=Vmin^(nq-2)/Vo^nq
  V1 : Inport  Port=1  LatchInput=off
  Math Function : Math  Operator=square  SaturateOnIntegerOverflow=on
  Mux2 : Mux  Inputs=2
  Mux3 : Mux  Inputs=2
  P0/ (Vo^np) : Gain  Gain=P0/(Mag_V0^np)  SaturateOnIntegerOverflow=on
  Q0/(Vo^nq) : Gain  Gain=Q0/(Mag_V0^nq)  SaturateOnIntegerOverflow=on
  Real-Imag to Complex : RealImagToComplex
  Switch3 : Switch  Threshold=Vmin  InputSameDT=on
  Switch4 : Switch  Threshold=Vmin  InputSameDT=on
  TF_P : Subsystem  mask(Transfer function){T1=Tp1, T2=Tp2, V_Init=P0}
      mask prompts: T1 "Time constant T1 (s):"; T2 "Time constant T2 (s):"; V_Init "Initial input and output :"
      mask help:
      | This block implements a continuous transfer function:
      |
      |          1+T1s
      | H(s)= ------
      |          1+T2s
      |
      | States are initialized according to  initial input and output value so that simulation starts in steady state.
      mask init:
      | numc=[T1 1];
      | denc=[T2 1];
      | [Ac,Bc,Cc,Dc]=tf2ss(numc,denc);
      | 
      | % Compute Initial states
      | I=eye(size(Ac));
      | x0c=inv(-Ac)*Bc*V_Init;
      mask Display: disp('1+T1s\n---\n1+T2s')
  TF_Q : Subsystem  mask(Transfer function){T1=Tq1, T2=Tq2, V_Init=Q0}
      mask prompts: T1 "Time constant T1 (s):"; T2 "Time constant T2 (s):"; V_Init "Initial input and output :"
      mask help:
      | This block implements a continuous transfer function:
      |
      |          1+T1s
      | H(s)= ------
      |          1+T2s
      |
      | States are initialized according to  initial input and output value so that simulation starts in steady state.
      mask init:
      | numc=[T1 1];
      | denc=[T2 1];
      | [Ac,Bc,Cc,Dc]=tf2ss(numc,denc);
      | 
      | % Compute Initial states
      | I=eye(size(Ac));
      | x0c=inv(-Ac)*Bc*V_Init;
      mask Display: disp('1+T1s\n---\n1+T2s')
  V^nq : Fcn  Expr=u[1]^u[2]
  V^nq , : Fcn  Expr=u[1]^u[2]
  Vmin^(np-2) : Gain  Gain=Vmin^(np-2)  SaturateOnIntegerOverflow=on
  Vmin^(nq-2) : Gain  Gain=Vmin^(nq-2)  SaturateOnIntegerOverflow=on
  np : Constant  Value=np
  nq : Constant  Value=nq
  P+jQ : Outport
  wires:
  Switch4/1 -> Q0/(Vo^nq)/1
  Real-Imag to Complex/1 -> P+jQ/1  "S_dyn=  P + j Q"
  P0/ (Vo^np)/1 -> TF_P/1(In1)
  Q0/(Vo^nq)/1 -> TF_Q/1(In1)
  Switch3/1 -> P0/ (Vo^np)/1
  np/1 -> Mux2/2
  Mux2/1 -> V^nq ,/1
  nq/1 -> Mux3/2
  Mux3/1 -> V^nq/1
  V1/1 -> Mux2/1, Mux3/1, Math Function/1, Switch3/2, Switch4/2
  V^nq/1 -> Switch4/1
  Math Function/1 -> Vmin^(np-2)/1, Vmin^(nq-2)/1
  Vmin^(np-2)/1 -> Switch3/3
  V^nq ,/1 -> Switch3/1
  Vmin^(nq-2)/1 -> Switch4/3
  TF_P/1(Out1) -> Real-Imag to Complex/1
  TF_Q/1(Out1) -> Real-Imag to Complex/2

== system powerlib_models/Phasors/asynchronous_machine/Negative Sequence Model ==
  note: Implementation of
      | V=RI+L.dI/dt  -> dI/dt= -(R/L)*I + V/L
      |
      | In dq components:
      | did/dt= w*(-r/l*id  +iq +vd/l)
      | diq/dt= w*(-r/l*iq -id + vq/l)
      | where r, l, i ,v are in pu
  Vqds2 : Inport  Port=1  LatchInput=off
  s2 : Inport  Port=2  LatchInput=off
  -pi/2  phase shift : Gain  Gain=exp(-j*pi/2)  SaturateOnIntegerOverflow=on
  Complex to Real-Imag : ComplexToRealImag
  Demux : Demux  Outputs=2
  Demux1 : Demux  Outputs=2
  Equivalent R2 L2 : Subsystem
  Gain1 : Gain  Gain=-1  SaturateOnIntegerOverflow=on
  Gain2 : Gain  Orientation=down  Gain=Rs  SaturateOnIntegerOverflow=on
  Gain3 : Gain  Orientation=left  Gain=[1 -1]  SaturateOnIntegerOverflow=on
  Gain4 : Gain  Gain=web_psb  SaturateOnIntegerOverflow=on
  Integrator : Integrator  InitialCondition=[0 0]
  Mux : Mux  Inputs=[1 1 2]
  Product1 : Product  Inputs=**  SaturateOnIntegerOverflow=on  InputSameDT=on
  Product2 : Product  Inputs=*/  SaturateOnIntegerOverflow=on  InputSameDT=on
  Product3 : Product  Inputs=**  SaturateOnIntegerOverflow=on  InputSameDT=on
  Real-Imag to Complex : RealImagToComplex
  Real-Imag to Complex1 : RealImagToComplex
  Selector1 : Selector  Orientation=left  Elements=[2 1]  InputPortWidth=2
  Sum : Sum  Inputs=+-+  SaturateOnIntegerOverflow=on  InputSameDT=on
  Sum1 : Sum  Orientation=down  Inputs=+-  SaturateOnIntegerOverflow=on  InputSameDT=on
  I2s : Outport
  I2r : Outport  Port=2
  Phiqds2_Iqds2 : Outport  Port=3
  wires:
  Real-Imag to Complex1/1 -> I2s/1, Product3/1, Gain2/1
  Demux1/2 -> Real-Imag to Complex1/1
  Demux1/1 -> Real-Imag to Complex1/2
  Gain1/1 -> I2r/1
  Product3/1 -> Gain1/1
  Equivalent R2 L2/3(Zm/(Zr+Zm)) -> Product3/2
  Equivalent R2 L2/1(L2_pu) -> Product2/2
  Product1/1 -> Sum/2  "Iqd2*R2/L2"
  Equivalent R2 L2/2(R2/L2_pu) -> Product1/2
  s2/1 -> Equivalent R2 L2/1(s2)
  Gain4/1 -> Integrator/1
  Sum/1 -> Gain4/1
  Product2/1 -> Sum/1  "Vqd2/L2"
  Integrator/1 -> Demux1/1, Product1/1, Gain3/1, Mux/3  "Iqds2"
  Gain3/1 -> Selector1/1
  Selector1/1 -> Sum/3  "[-id2 iq2]"
  Vqds2/1 -> Product2/1, Demux/1
  Demux/1 -> Real-Imag to Complex/2
  Demux/2 -> Real-Imag to Complex/1
  Gain2/1 -> Sum1/2
  Sum1/1 -> -pi/2  phase shift/1  "Vm2"
  -pi/2  phase shift/1 -> Complex to Real-Imag/1  "Phi2"
  Real-Imag to Complex/1 -> Sum1/1
  Complex to Real-Imag/2 -> Mux/1  "Phiqs2"
  Mux/1 -> Phiqds2_Iqds2/1
  Complex to Real-Imag/1 -> Mux/2  "Phids2"

== system powerlib_models/Phasors/asynchronous_machine/Positive Sequence Model ==
  Vqdr1 : Inport  Port=1  LatchInput=off
  w-wr : Inport  Port=2  LatchInput=off
  Vqds1 : Inport  Port=3  LatchInput=off
  Constant7 : Constant
  Mutual fluxes : Subsystem  Orientation=left
  Rotor : Subsystem
      mask Display: disp('Rotor')
  Stator : Subsystem
      mask Display: disp('Stator')
  Iqdr1 : Outport
  phiqdr1 : Outport  Port=2
  phiqds1 : Outport  Port=3
  Iqds1 : Outport  Port=4
  Phiqds1_Isqds1 : Outport  Port=5
  wires:
  Stator/3(phis,is) -> Phiqds1_Isqds1/1
  Stator/2(iqs,ids) -> Iqds1/1
  w-wr/1 -> Rotor/2(w-wr)
  Rotor/1(iqr,idr) -> Iqdr1/1
  Vqds1/1 -> Stator/2(vqs,vds)
  Vqdr1/1 -> Rotor/1(vqr,vdr)
  Constant7/1 -> Stator/3(w)
  Rotor/2(phiqr,phidr) -> phiqdr1/1, Mutual fluxes/1(phiqr,phidr)
  Stator/1(phiqs,phids) -> phiqds1/1, Mutual fluxes/2(phiqs,phids)
  Mutual fluxes/1(phimq,phimd) -> Rotor/3(phimq,phimd), Stator/1(phimq,phimd)

== system powerlib_models/Phasors/asynchronous_machine/abc2dq ==
  note: V2= 1/3(Vab -a*Vbc)
  note: V1= 1/3(Vab -a^2*Vbc)
  Vab Vbc cmplx : Inport  Port=1  LatchInput=off
  (a^2)/3 : Gain  Gain=1/3*exp(-j*2*pi/3)  SaturateOnIntegerOverflow=on
  Complex to Real-Imag : ComplexToRealImag
  Complex to Real-Imag3 : ComplexToRealImag
  Demux : Demux  Outputs=2
  Gain : Gain  Gain=1/3  SaturateOnIntegerOverflow=on
  Gain1 : Gain  Gain=1/3  SaturateOnIntegerOverflow=on
  Mux : Mux  Inputs=2
  Mux3 : Mux  Inputs=2
  Sum3 : Sum  Inputs=+-  SaturateOnIntegerOverflow=on  InputSameDT=on
  Sum4 : Sum  Inputs=+-  SaturateOnIntegerOverflow=on  InputSameDT=on
  a/3 : Gain  Gain=1/3*exp(j*2*pi/3)  SaturateOnIntegerOverflow=on
  Vqds1 : Outport
  Vqds2 : Outport  Port=2
  wires:
  Mux3/1 -> Vqds2/1
  Complex to Real-Imag3/1 -> Mux3/2
  Complex to Real-Imag3/2 -> Mux3/1
  Sum4/1 -> Complex to Real-Imag3/1  "V2"
  (a^2)/3/1 -> Sum3/2
  Demux/2 -> (a^2)/3/1, a/3/1
  Gain/1 -> Sum3/1
  Vab Vbc cmplx/1 -> Demux/1
  Gain1/1 -> Sum4/1
  a/3/1 -> Sum4/2
  Demux/1 -> Gain/1, Gain1/1
  Sum3/1 -> Complex to Real-Imag/1  "V1"
  Complex to Real-Imag/1 -> Mux/2
  Complex to Real-Imag/2 -> Mux/1
  Mux/1 -> Vqds1/1

== system powerlib_models/Phasors/asynchronous_machine/dq2abc ==
  iqdr1 : Inport  Port=1  LatchInput=off
  iqds1 : Inport  Port=2  LatchInput=off
  Ir2 : Inport  Port=3  LatchInput=off
  Is2 : Inport  Port=4  LatchInput=off
  Phasors Ia Ib rotor : Subsystem
  Phasors Ia Ib stator : Subsystem
  irabc : Outport
  isabc : Outport  Port=2
  wires:
  Is2/1 -> Phasors Ia Ib stator/2(I2s)
  Ir2/1 -> Phasors Ia Ib rotor/2(I2r)
  Phasors Ia Ib rotor/1(Irabc cmplx) -> irabc/1
  Phasors Ia Ib stator/1(Isabc cmplx) -> isabc/1
  iqdr1/1 -> Phasors Ia Ib rotor/1(Iqdr1)
  iqds1/1 -> Phasors Ia Ib stator/1(Iqds1)
